simulink model "LateralModelErrorControl"  (R2020b)
settings: Solver=FixedStepAuto  StartTime=0.0  StopTime=400  FixedStep=0.01  RelTol=1e-3
InitFcn:
  | load('waypoints.mat');
  | VehicleObj = Simulink.data.dictionary.open('VehicleData.sldd');
  | %dDataSectObj = getSection(myDictionaryObj,'Design Data');
StopFcn:
  | Plot_LateralModelErrorControl;
values from neighbouring files (symbols this model uses):
  C_af = 80000.0    [VehicleData.sldd]
  C_ar = 80000.0    [VehicleData.sldd]
  g = 9.81    [VehicleData.sldd]
  Iz = 2873.0    [VehicleData.sldd]
  lf = 1.1    [VehicleData.sldd]
  lr = 1.58    [VehicleData.sldd]
  m = 2238.932    [VehicleData.sldd]
settings Model: DataDictionary=VehicleData.sldd  Creator=headl  LastModifiedBy=uidv8616
settings DataIOCC: ReturnWorkspaceOutputs=off  DSMLoggingName=datalog
settings DebuggingCC: SignalRangeChecking=warning
settings SFSimCC: CustomCodeUndefinedFunction=UseInterfaceOnly

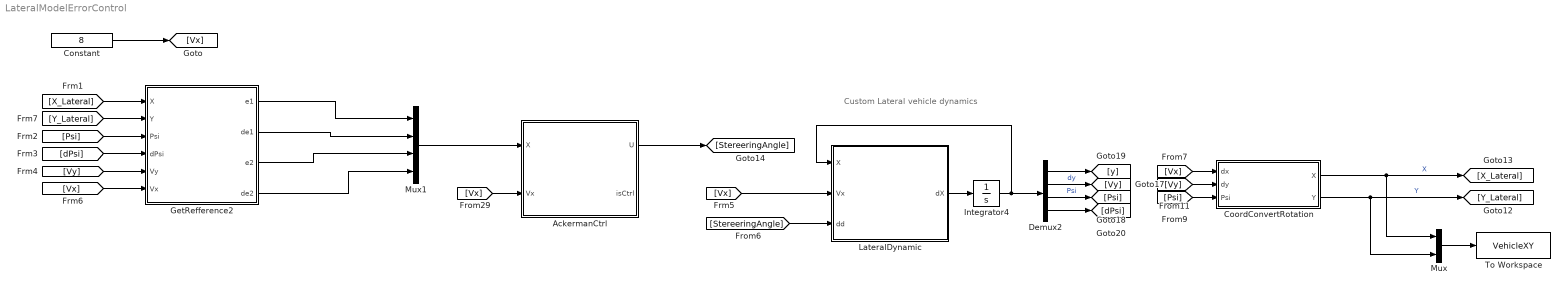
== system LateralModelErrorControl ==
  note: Custom Lateral vehicle dynamics
  AckermanCtrl : MATLAB Function  TreatAsAtomicUnit=on
  Constant : Constant  Value=8
  CoordConvertRotation : Subsystem
  Demux2 : Demux
  GetRefference2 : MATLAB Function  TreatAsAtomicUnit=on
  Integrator4 : Integrator  InitialCondition=[0;0;-1.574;0.0423]
  LateralDynamic : MATLAB Function  TreatAsAtomicUnit=on
  Mux : Mux  Inputs=2
  Mux1 : Mux
  To Workspace : ToWorkspace  VariableName=VehicleXY  SampleTime=-1
  wires:
  Constant/1 -> [Vx]
  Demux2/1 -> [y]
  LateralDynamic/1(dX) -> Integrator4/1
  [Vx] -> CoordConvertRotation/1(dx)
  Integrator4/1 -> Demux2/1, LateralDynamic/1(X)
  [Vy] -> CoordConvertRotation/2(dy)
  Demux2/2 -> [Vy]  "dy"
  Demux2/4 -> [dPsi]
  Demux2/3 -> [Psi]  "Psi"
  [StereeringAngle] -> LateralDynamic/3(dd)
  [Vx] -> LateralDynamic/2(Vx)
  [Psi] -> CoordConvertRotation/3(Psi)
  CoordConvertRotation/2(Y) -> Mux/2, [Y_Lateral]  "Y"
  CoordConvertRotation/1(X) -> Mux/1, [X_Lateral]  "X"
  [Vx] -> AckermanCtrl/2(Vx)
  Mux1/1 -> AckermanCtrl/1(X)
  Mux/1 -> To Workspace/1
  [X_Lateral] -> GetRefference2/1(X)
  [Y_Lateral] -> GetRefference2/2(Y)
  [Psi] -> GetRefference2/3(Psi)
  [dPsi] -> GetRefference2/4(dPsi)
  [Vy] -> GetRefference2/5(Vy)
  [Vx] -> GetRefference2/6(Vx)
  GetRefference2/1(e1) -> Mux1/1
  GetRefference2/2(de1) -> Mux1/2
  GetRefference2/3(e2) -> Mux1/3
  GetRefference2/4(de2) -> Mux1/4
  AckermanCtrl/1(U) -> [StereeringAngle]

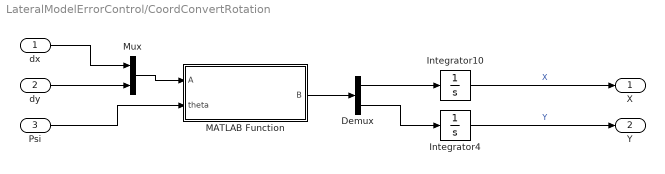
== system LateralModelErrorControl/CoordConvertRotation ==
  dx : Inport
  dy : Inport  Port=2
  Psi : Inport  Port=3
  Demux : Demux  Outputs=2
  Integrator10 : Integrator  InitialCondition=-181.34188
  Integrator4 : Integrator  InitialCondition=78.53502
  MATLAB Function : MATLAB Function  TreatAsAtomicUnit=on
  Mux : Mux  Inputs=2
  X : Outport  VectorParamsAs1DForOutWhenUnconnected=off
  Y : Outport  Port=2  VectorParamsAs1DForOutWhenUnconnected=off
  wires:
  Integrator10/1 -> X/1  "X"
  Integrator4/1 -> Y/1  "Y"
  Psi/1 -> MATLAB Function/2(theta)
  dx/1 -> Mux/1
  dy/1 -> Mux/2
  Mux/1 -> MATLAB Function/1(A)
  MATLAB Function/1(B) -> Demux/1
  Demux/1 -> Integrator10/1
  Demux/2 -> Integrator4/1

== matlab function LateralModelErrorControl/CoordConvertRotation/MATLAB Function ==
  data: A input; B output; theta input
function B = RotateVector(A, theta)
B = [0;0];
R = [cos(theta) -sin(theta); sin(theta) cos(theta)];

B = R*A;

== matlab function LateralModelErrorControl/GetRefference2 ==
  data: e1 output size=1; X input size=1; Y input double size=1; racetrackwaypoints parameter; de1 output; e2 output; de2 output; Psi input; dPsi input; Vy input; Vx input
function [e1,de1,e2,de2] = GetReff(X,Y,racetrackwaypoints, Psi,dPsi, Vy, Vx) 

PQ = [X,Y]; % current Intertial position of vehicle
P = racetrackwaypoints(:,1:2); % List of waypoints column1 = X coord.  column2 = Y coord.
[k,D] = knnsearch(P,PQ); % locate the closest waypoint to the vehicle. k = index, D = distance
k = k(1);


% here I take 3 points: the closest, one behind, one in front.
P_road1 = P(k-1,:);
P_road2 = P(k,:);
P_road3 = P(k+1,:);

F = atan2( (P(k+5,2)-P(k,2)),(P(k+5,1)-P(k,1))); % Obtaining the road orientation
psi_des = F(1);

P_veh = PQ - P_road2;

%B = [P(k,1);P(k,2)];
% Convert from intertial coordinates system to body fixed system. C.G. as
% center and rotated Psi degrees.
M_Rot = [cos(psi_des) -sin(psi_des); sin(psi_des) cos(psi_des)];
P_road1 = (P_road1-P_road2)*M_Rot;
P_road2 = (P_road2-P_road2)*M_Rot;
P_road3 = (P_road3-P_road2)*M_Rot;
P_veh = P_veh*M_Rot;



%e1 = X-P_veh2(1);
e1 = P_veh(2); % error e1



e2 = Psi - psi_des; % error e2

de1 = Vy + Vx*(e2); % derivative of e1


% Obtainig the radius of imaginary circle of the curve
Xc = [P_road1(1);P_road2(1);P_road3(1)];
Yc = [P_road1(2);P_road2(2);P_road3(2)];

% Xc = [P(k-1,1);P(k,1);P(k+1,1)];
% Yc = [P(k-1,2);P(k,2);P(k+1,2)];
[xc,yc,R,a] = circfit(Xc,Yc);
% R = R *  sign(P(k,1)-xc);
R = R*sign(yc);


%in streight line, the radius falls into singularity. here is detected
%and solved with a minimum
eval = ~isfinite(R);
if eval
 R = 100000;   
end

dPsi_des = Vx/R; % derivative of orientation refference
de2 = dPsi - dPsi_des; % derivative of e2

end

== matlab function LateralModelErrorControl/LateralDynamic ==
  data: dX output; X input; Vx input; dd input; C_af parameter; C_ar parameter; lf parameter; lr parameter; Iz parameter; m parameter
%*****************************************************
% BICYCLE MODEL OF LATERAL VEHICLE DYNAMICS
% Taken from Rajamani chapter 2.3 page 30
function dX = bicycleModelOde(X,Vx,dd, C_af, C_ar, lf, lr, Iz, m) % pd polos deseados
dX = [0;0;0;0];
y = X(1);
dy = X(2);
Psi = X(3);
dPsi = X(4);


A22 = -(2*C_af+2*C_ar)/(m*Vx);
A24 = -Vx- (2*C_af*lf-2*C_ar*lr)/(m*Vx);
A42 = -(2*lf*C_af-2*lr*C_ar)/(Iz*Vx);
A44 = -(2*lf^2*C_af + 2*lr^2*C_ar)/(Iz*Vx);

B21 = 2*C_af/m;
B41 = 2*lf*C_af/Iz;

A = [0 1 0 0;0 A22 0 A24;0 0 0 1;0 A42 0 A44];
B = [0;B21;0;B41];

dX= A*X(1:4) + B*dd; 

end

== matlab function LateralModelErrorControl/AckermanCtrl ==
  data: U output size=1; X input; Vx input; isCtrl output; C_af parameter; g parameter; C_ar parameter; lf parameter; lr parameter; Iz parameter; m parameter
% ******************* Lateral dynamic controller *********************
%*********************************************************************
% Author: L.Arturo Torres-Romero
% Date: 22-10-2020
% This controller controlls the direction of a car, based in the dynamics
% described  in the next link and using the Ackerman formulation: 
% https://www.researchgate.net/publication/340166902_LATERAL_VEHICLE_DYNAMICS_AND_CONTROLLERS_DESIGN


%******************* PARAMETERS DESCRIPTIONS **********************
%******************************************************************
% m: vehicle mass
% g: gravity
% C_af : Cornering  stiffness  of  front  wheels.
% C_ar : Cornering  stiffness  of  rear  wheels.
% lf : distance fron the center of gravity to the front wheel axis.
% lr : distance fron the center of gravity to the rear wheel axis.
% Iz : this is the momentum of inertia of the vehicle respect the z axis.
%******************************************************************
%******************* INPUTS DESCRIPTIONS **************************
%******************************************************************
% X:   (column vector)[e1;de1;e2;de2] states of the state space of 
%       the system that includes the errors as follows:
%      e1  : is the lateral position error respect the road.
%      de1 : derivative of e1.
%      e2  : is the yaw angle error with respect the road. 
%      de2 : derivarive of the e2.

% Vx: Logitudinal velocity.



%******************************************************************
% ******************* OUTPUTS DESCRIPTIONS ************************
%******************************************************************
% U: control coutput in radians. Angle of the frontal wheels respect to the
%    longitudinal axis
% isCtrl: when true means that the matrix Mc has full rank, and hence, the
%         system is controllable


%******************************************************************


function [U,isCtrl] = AckermanLateralCtrl(X, Vx, C_af, g, C_ar, lf, lr, Iz, m) % pd polos deseados

%**************************************************
%******* Matrix A formulation *********************
A22 = -(2*C_af + 2*C_ar)/(m*Vx);
A23 = (2*C_af + 2*C_ar)/m;
A24 = (-2*C_af*lf + 2*C_ar*lr)/(m*Vx);
A42 = -(2*C_af*lf - 2*C_ar*lr)/(Iz*Vx);
A43 = (2*C_af*lf - 2*C_ar*lr)/Iz;
A44 = -(2*C_af*lf^2 + 2*C_ar*lr^2)/(Iz*Vx);

A = [0 1 0 0;0 A22 A23 A24;0 0 0 1;0 A42 A43 A44];
%**************************************************

%**************************************************
%******* Matrix B1 formulation ********************
B1_2 = 2*C_af/m;
B1_4 = 2*C_af*lf/Iz;

B1 = [0;B1_2;0;B1_4];
%***************************************************

%***************************************************
%******* Matrix B2 formulation *********************
B2_2 = -(2*C_af*lf - 2*C_ar*lr)/(m*Vx) - Vx;
B2_4 = -(2*C_af*lf^2 + 2*C_ar*lr^2)/(Iz*Vx);

B2 = [0;B2_2;0;B2_4];
%***************************************************


%***************************************************
%******* Matrix B3 formulation *********************
B3 = [0;g;0;0];
%***************************************************


%***************************************************
%******* Verification of controllability and output 
% calculation of the controller
%**************************************************
ctrlVal = 0;
Mc = [B1 A*B1 A^2*B1 A^3*B1];
rankVal = rank(Mc);
    if rankVal < size(A,1)
        %disp('Not completely state controllable');
        isCtrl = 0;
        ctrlVal = 0;
    else
        %disp('Completely state controllable');
        isCtrl = 1;
        % Pole placement
        Pd =[-5-3i -5+3i -7 -10];
        %Pd =[-2 -2 -2 -2];

        H = (A- Pd(1)*eye(4)) * (A- Pd(2)*eye(4)) * (A- Pd(3)*eye(4)) * (A- Pd(4)*eye(4));

        %ackerman formula
        K = [0 0 0 1]*Mc^-1*H;
        ctrlVal = -K*X;  
    end


U = real(ctrlVal);
